simulink model "Ex3_1_sim"  (R2015a)
settings: Solver=ode45  StartTime=0.0  StopTime=60.0  RelTol=1e-3
values from neighbouring files (symbols this model uses):
  K = R    (= 0.8)    [Ex3_1.m]
  q1 = 0.5    [Ex3_1.m]
  T = A*R    (= 8)    [Ex3_1.m]
settings Model: CovSFcnEnable=off  Creator=Shin  LastModifiedBy=Shin
settings DebuggingCC: SolverPrmCheckMsg=warning

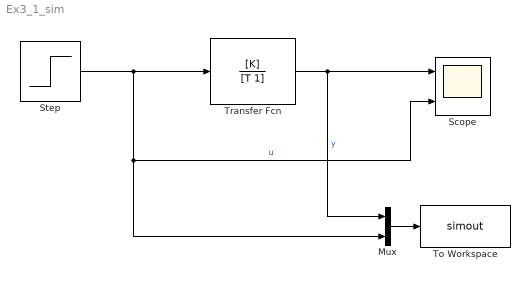
== system Ex3_1_sim ==
  Mux : Mux  Inputs=2
  Scope : Scope  NumInputPorts=2
      settings: YMin=0~0  YMax=0.5~1
  Step : Step  After=q1  SampleTime=0
  To Workspace : ToWorkspace  VariableName=simout  SaveFormat=Timeseries  SampleTime=-1
  Transfer Fcn : TransferFcn  Numerator=[K]  Denominator=[T 1]
  wires:
  Transfer Fcn/1 -> Mux/1, Scope/1  "y"
  Step/1 -> Mux/2, Scope/2, Transfer Fcn/1  "u"
  Mux/1 -> To Workspace/1
